simulink model "boucle_fermee_reduite_13_10_2025"  (R2025a)
settings: Solver=VariableStepAuto  StartTime=0.0  StopTime=0.1  FixedStep=1e-4  RelTol=1e-3
undefined symbols (not defined in the file): f, J, Kphi, L, R, Rch, U1
settings Model: Creator=ltroullier01  LastModifiedBy=etrenchant01

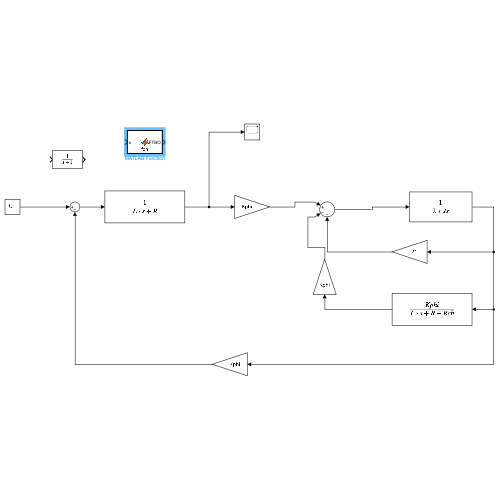
[thumbnail: Simulink's stored preview of the top-level diagram]
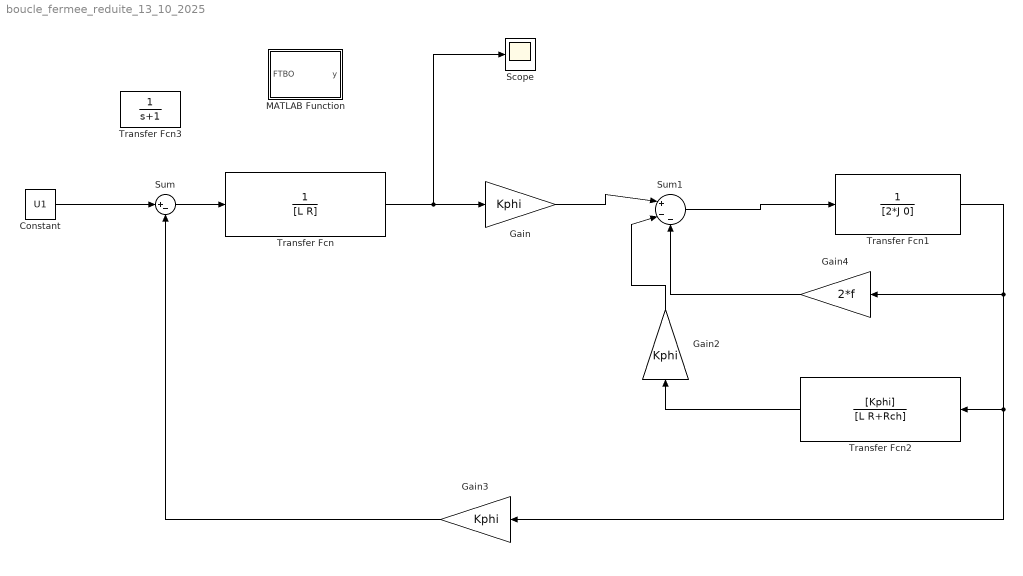
== system boucle_fermee_reduite_13_10_2025 ==
  Constant : Constant  Value=U1
  Gain : Gain  Gain=Kphi
  Gain2 : Gain  Gain=Kphi
  Gain3 : Gain  Gain=Kphi
  Gain4 : Gain  Gain=2*f
  MATLAB Function : MATLAB Function  TreatAsAtomicUnit=on
  Scope : Scope
      settings: ActiveDisplayYMinimum=-4.9369832712561159  ActiveDisplayYMaximum=31.373841687864346
  Sum : Sum  Inputs=|+-
  Sum1 : Sum  Inputs=|+--
  Transfer Fcn : TransferFcn  Denominator=[L R]
  Transfer Fcn1 : TransferFcn  Denominator=[2*J 0]
  Transfer Fcn2 : TransferFcn  Numerator=[Kphi]  Denominator=[L R+Rch]
  Transfer Fcn3 : TransferFcn  Denominator=[1 1]
  wires:
  Constant/1 -> Sum/1
  Sum/1 -> Transfer Fcn/1
  Transfer Fcn1/1 -> Gain3/1, Transfer Fcn2/1, Gain4/1
  Transfer Fcn/1 -> Scope/1, Gain/1
  Gain/1 -> Sum1/1
  Sum1/1 -> Transfer Fcn1/1
  Transfer Fcn2/1 -> Gain2/1
  Gain3/1 -> Sum/2
  Gain2/1 -> Sum1/2
  Gain4/1 -> Sum1/3

== matlab function boucle_fermee_reduite_13_10_2025/MATLAB Function ==
  data: FTBO input; y output
function y = fcn(FTBO)

y = FTBO;
